simulink model "sim_ekf_est_all_para_v3"  (R2021b)
settings: Solver=FixedStepAuto  StartTime=0.0  StopTime=60  FixedStep=0.01  RelTol=1e-3
settings Model: Creator=Admin  LastModifiedBy=ASUS
settings SolverCC: AlgebraicLoopSolver=TrustRegion
settings DebuggingCC: SFMachineParentedDataDiag=warning

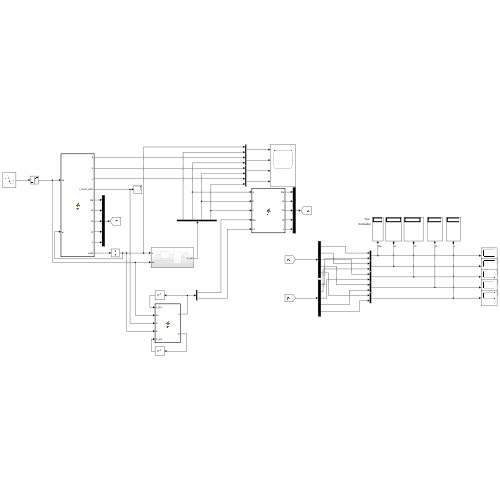
[thumbnail: Simulink's stored preview of the top-level diagram]
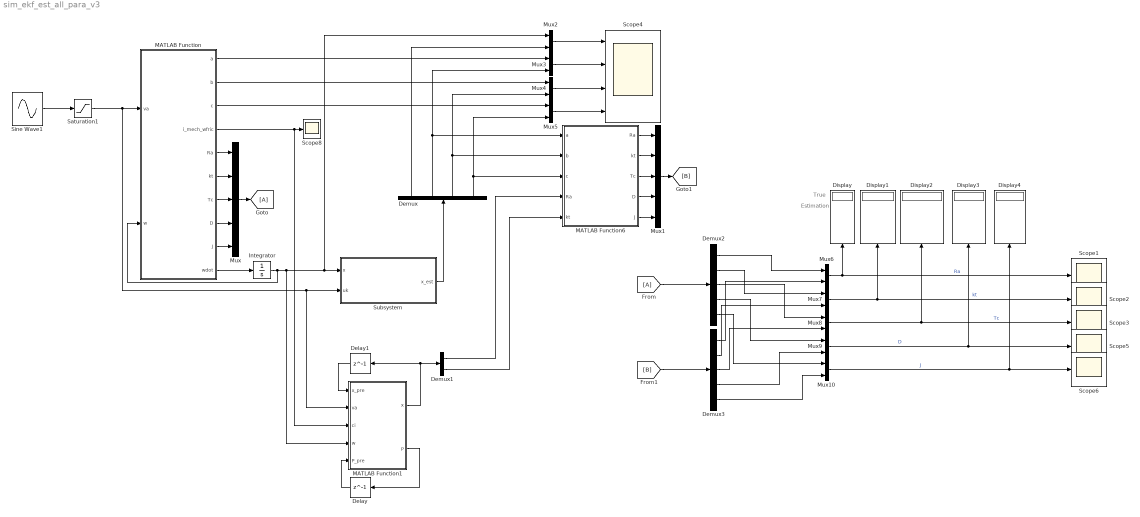
== system sim_ekf_est_all_para_v3 ==
  note: Estimation
  note: True
  Delay : Delay  DelayLength=1  InitialCondition=diag([5,0.1])
  Delay1 : Delay  DelayLength=1  InitialCondition=[5;0]
  Demux : Demux
  Demux1 : Demux  Outputs=2
  Demux2 : Demux  Outputs=5
  Demux3 : Demux  Outputs=5
  Display{,1..4} (5 alike) : Display
  Integrator : Integrator
  MATLAB Function : MATLAB Function  TreatAsAtomicUnit=on
  MATLAB Function1 : MATLAB Function  TreatAsAtomicUnit=on
  MATLAB Function6 : MATLAB Function  TreatAsAtomicUnit=on
  Mux : Mux  Inputs=5
  Mux1 : Mux  Inputs=5
  Mux{2..10} (9 alike) : Mux  Inputs=2
  Saturation1 : Saturate  UpperLimit=24  LowerLimit=-24
  Scope{1..3,5..6,8} (6 alike) : Scope
  Scope4 : Scope  NumInputPorts=4
  Sine Wave1 : Sin  Amplitude=10  Frequency=2*pi*0.1  SampleTime=0
  Subsystem : Subsystem
  wires:
  MATLAB Function/2(b) -> Mux4/1
  Sine Wave1/1 -> Saturation1/1
  Saturation1/1 -> MATLAB Function1/2(va), Subsystem/2(uk), MATLAB Function/1(va)
  MATLAB Function/3(c) -> Mux5/1
  MATLAB Function/10(wdot) -> Integrator/1
  MATLAB Function/1(a) -> Mux3/1
  Integrator/1 -> Subsystem/1(x), Mux2/1, MATLAB Function1/4(w), MATLAB Function/2(w)
  Mux2/1 -> Scope4/1
  Mux3/1 -> Scope4/2
  Mux4/1 -> Scope4/3
  Mux5/1 -> Scope4/4
  Demux/1 -> Mux2/2
  Demux/2 -> Mux3/2, MATLAB Function6/1(a)
  Demux/3 -> Mux4/2, MATLAB Function6/2(b)
  Demux/4 -> Mux5/2, MATLAB Function6/3(c)
  Subsystem/1(x_est) -> Demux/1
  MATLAB Function/5(Ra) -> Mux/1
  MATLAB Function/6(kt) -> Mux/2
  MATLAB Function/7(Tc) -> Mux/3
  MATLAB Function/8(D) -> Mux/4
  MATLAB Function/9(J) -> Mux/5
  MATLAB Function6/1(Ra) -> Mux1/1
  MATLAB Function6/2(kt) -> Mux1/2
  MATLAB Function6/3(Tc) -> Mux1/3
  MATLAB Function6/4(D) -> Mux1/4
  MATLAB Function6/5(J) -> Mux1/5
  Mux/1 -> [A]
  Mux1/1 -> [B]
  Mux6/1 -> Display/1, Scope1/1  "Ra"
  Mux7/1 -> Display1/1, Scope2/1  "kt"
  Mux8/1 -> Scope3/1, Display2/1  "Tc"
  Mux9/1 -> Display3/1, Scope5/1  "D"
  Mux10/1 -> Display4/1, Scope6/1  "J"
  [A] -> Demux2/1
  [B] -> Demux3/1
  Demux2/1 -> Mux6/1
  Demux2/2 -> Mux7/1
  Demux2/3 -> Mux8/1
  Demux2/4 -> Mux9/1
  Demux2/5 -> Mux10/1
  Demux3/1 -> Mux6/2
  Demux3/2 -> Mux7/2
  Demux3/3 -> Mux8/2
  Demux3/4 -> Mux9/2
  Demux3/5 -> Mux10/2
  Delay1/1 -> MATLAB Function1/1(x_pre)
  Delay/1 -> MATLAB Function1/5(P_pre)
  MATLAB Function1/1(x) -> Delay1/1, Demux1/1
  MATLAB Function1/2(P) -> Delay/1
  MATLAB Function/4(i_mech_wfric) -> MATLAB Function1/3(ci), Scope8/1
  Demux1/1 -> MATLAB Function6/4("Ra ")
  Demux1/2 -> MATLAB Function6/5("kt ")

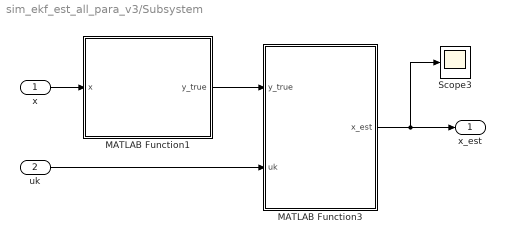
== system sim_ekf_est_all_para_v3/Subsystem ==
  x : Inport
  uk : Inport  Port=2
  MATLAB Function1 : MATLAB Function  TreatAsAtomicUnit=on
  MATLAB Function3 : MATLAB Function  TreatAsAtomicUnit=on
  Scope3 : Scope
  x_est : Outport
  wires:
  MATLAB Function1/1(y_true) -> MATLAB Function3/1(y_true)
  MATLAB Function3/1(x_est) -> Scope3/1, x_est/1
  uk/1 -> MATLAB Function3/2(uk)
  x/1 -> MATLAB Function1/1(x)

== matlab function sim_ekf_est_all_para_v3/Subsystem/MATLAB Function1 ==
  settings: updateMethod=DISCRETE
  data: x input; y_true output
function y_true = output_eq(x)
x = [x;0;0;0];
C = [1 0 0 0];
y_true = C*x+sqrt(0.001)*randn;

== matlab function sim_ekf_est_all_para_v3/MATLAB Function ==
  settings: updateMethod=DISCRETE
  data: a output; b output; c output; i_mech_wfric output; Ra output; kt output; Tc output; D output; J output; va input; wdot output; w input
function [a,b,c,i_mech_wfric,Ra,kt,Tc,D,J,wdot] = fcn(va,w)
%parameters from datasheet
Ra = 14.3;
kt = 0.05; %kb = 0.063;
kb = kt;
Tc = 0.053*kt;
D  = 9.4e-5*kt;
J = 1.94e-4*kt;

% lumped parameters
a = ((kb*kt+D*Ra)/(Ra*J));
b = (kt/(Ra*J));
c = (Tc/J);

% model
wdot = -a*w + b*va - c*sign(w);

% i_elec = (va - kb*w)/Ra;
% i_mech_nfric = (D*w + J*wdot)/kt;
i_mech_wfric = (Tc*sign(w)+0.001*randn+D*w + J*wdot)/kt;

== matlab function sim_ekf_est_all_para_v3/Subsystem/MATLAB Function3 ==
  settings: updateMethod=DISCRETE
  data: y_true input; x_est output; uk input
function x_est = ekf(y_true, uk)
Ts = 0.01;
persistent x_est_p P Qd_est R_est Qc_est;
if isempty(x_est_p)
    x_est_p = [0;0;0;0];
    P       = 1e0*diag([10,1,30,10]);
    Qc_est  = 1e-4*diag([1,10,100,10]);
    Qd_est  = Ts*Qc_est;
    R_est   = 0.01;
end
c  = [1 0 0 0];
D  = 0;
Ck = c;
Dk = D;

%Comput Kalman Gain and update predicted value
Wk    = P*Ck'/(Ck*P*Ck'+R_est);
y_est = Ck*x_est_p+Dk*uk;
x     = x_est_p+Wk.*(y_true-y_est);

%Compute prediction at next time step
x_est = x+Ts*[-x(2)*x(1)+uk*x(3)-x(4)*sign(x(1));
    0;
    0;
    0];

%Update error covariance matrices
P = P-Wk*Ck*P;

%Define Ak
Ak      = eye(4)+Ts*[-x(2) -x(1) uk -sign(x(1));
    0     0    0      0;
    0     0    0      0;
    0     0    0      0];
P       = Ak*P*Ak'+Qd_est;
x_est_p = x_est;

== matlab function sim_ekf_est_all_para_v3/MATLAB Function1 ==
  data: x_pre input; va input; ci input; w input; P_pre input; x output; P output
function [x,P] = fcn(x_pre,va,ci,w,P_pre)
% Initialize step, putted in the delay instead
% P = (A'A)^-1;
% x = P*(A'b);

% calculate state
A = [1 w/ci];
b = va/ci;

% recursive least square method
P = P_pre - P_pre*A'/(1+A*P_pre*A')*(A*P_pre);
K = P*A';
x = x_pre + K*(b-A*x_pre);

== matlab function sim_ekf_est_all_para_v3/MATLAB Function6 ==
  data: Ra output; kt output; Tc output; D output; a input; b input; c input; Ra input; J output; kt input
function [Ra,kt,Tc,D,J] = fcn(a,b,c,Ra,kt)
Ra = Ra;
kt = kt;

J = (kt/(Ra*b));
Tc = (c*J);
D = (a*Ra*J - kt^2)/Ra;
